simulink model "Trajectory"  (R2025a)
settings: Solver=VariableStepAuto  StartTime=0.0  StopTime=65  FixedStep=0.01  RelTol=1e-3
values from neighbouring files (symbols this model uses):
  L = 0.2    [untitled2.m]
  P = densifyPath(path, 0.05)    [untitled2.m]
  start = [1 1]    [untitled2.m]
undefined symbols (not defined in the file or in its folder): Actor, createShape
libraries: slpidlib x2, sim3dlib x2, robotalgslib x1
settings Model: Creator=mwali  LastModifiedBy=mwali

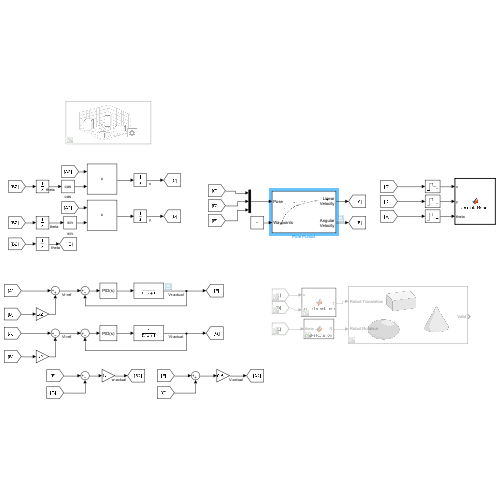
[thumbnail: Simulink's stored preview of the top-level diagram]
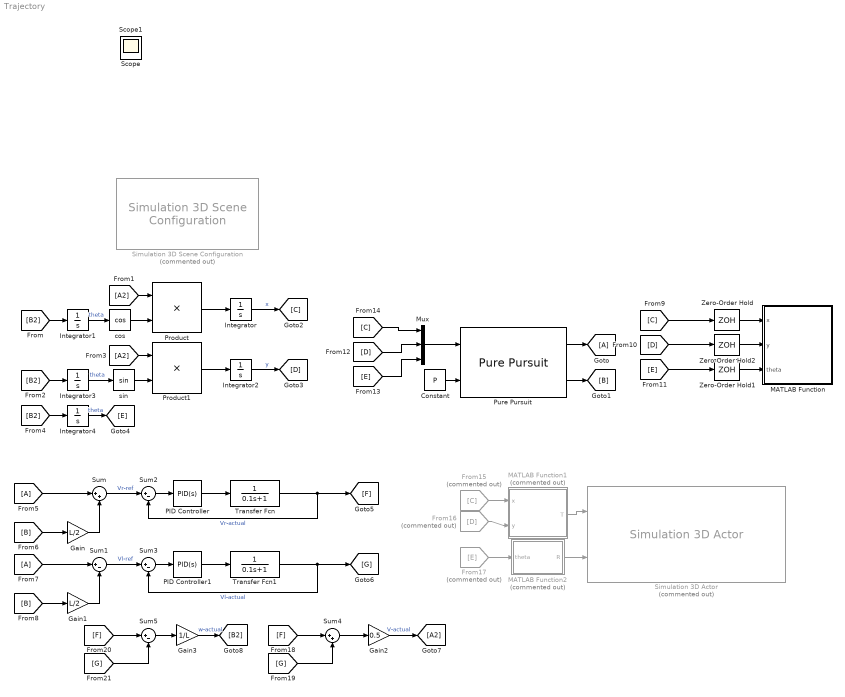
== system Trajectory ==
  Constant : Constant  Value=P
  From15 : From  Commented=on  GotoTag=C
  From16 : From  Commented=on  GotoTag=D
  From17 : From  Commented=on  GotoTag=E
  From5 : From
  From7 : From
  Gain : Gain  Gain=L/2
  Gain1 : Gain  Gain=L/2
  Gain2 : Gain  Gain=0.5
  Gain3 : Gain  Gain=1/L
  Goto : Goto
  Integrator : Integrator  InitialCondition=start(1)
  Integrator1 : Integrator
  Integrator2 : Integrator  InitialCondition=start(2)
  Integrator3 : Integrator
  Integrator4 : Integrator
  MATLAB Function : MATLAB Function  TreatAsAtomicUnit=on
  MATLAB Function1 : MATLAB Function  Commented=on  TreatAsAtomicUnit=on
  MATLAB Function2 : MATLAB Function  Commented=on  TreatAsAtomicUnit=on
  Mux : Mux  Inputs=3
  PID Controller : slpidlib/PID Controller  Controller=PID  Form=Parallel  TimeDomain=Continuous-time  UseExternalTs=off  SampleTime=-1  IntegratorMethod=Forward Euler  FilterMethod=Forward Euler  ControllerParametersSource=internal  P=1.08351767141455  I=20.5811272107881  UseKiTs=off  D=-0.0128072394159001  UseExternalDerivativeSource=off  N=84.6019689511989  UseFilter=on  TunerSelectOption=Transfer Function Based (PID Tuner App)  InitialConditionSource=internal  InitialConditionForIntegrator=0  InitialConditionForFilter=0  DifferentiatorICPrevScaledInput=0  ExternalReset=none  TrackingMode=off  Kt=1  LimitOutput=off  SatLimitsSource=internal  UpperSaturationLimit=inf  LowerSaturationLimit=-inf  LinearizeAsGain=on  AntiWindupMode=none  Kb=1  LimitIntegrator=off  UpperIntegratorSaturationLimit=inf  LowerIntegratorSaturationLimit=-inf  POutMin=[]  POutMax=[]  IOutMin=[]  IOutMax=[]  DOutMin=[]  DOutMax=[]  NOutMin=[]  NOutMax=[]  SumOutMin=[]  SumOutMax=[]  SaturationOutMin=[]  SaturationOutMax=[]  PParamMin=[]  PParamMax=[]  IParamMin=[]  IParamMax=[]  DParamMin=[]  DParamMax=[]  NParamMin=[]  NParamMax=[]  KbParamMin=[]  KbParamMax=[]  KtParamMin=[]  KtParamMax=[]  KbOutMin=[]  KbOutMax=[]  KtOutMin=[]  KtOutMax=[]  IntegratorOutMin=[]  IntegratorOutMax=[]  FilterOutMin=[]  FilterOutMax=[]  SumI1OutMin=[]  SumI1OutMax=[]  SumI2OutMin=[]  SumI2OutMax=[]  SumI3OutMin=[]  SumI3OutMax=[]  SumI4OutMin=[]  SumI4OutMax=[]  SumDOutMin=[]  SumDOutMax=[]  DifferentiatorOutMin=[]  DifferentiatorOutMax=[]  FilterDiffOutCoefMin=[]  FilterDiffOutCoefMax=[]  ReciprocalOutMin=[]  ReciprocalOutMax=[]  SumDenOutMin=[]  SumDenOutMax=[]  SumNumOutMin=[]  SumNumOutMax=[]  DivideOutMin=[]  DivideOutMax=[]  UdiffTsProdOutMin=[]  UdiffTsProdOutMax=[]  NTsProdOutMin=[]  NTsProdOutMax=[]  UintegralTsProdOutMin=[]  UintegralTsProdOutMax=[]  UngainTsProdOutMin=[]  UngainTsProdOutMax=[]  ClampingZeroOutDataTypeStr=Inherit: Inherit via back propagation  ClampingZeroOutMin=[]  ClampingZeroOutMax=[]  FilterDenConstantOutDataTypeStr=Inherit: Inherit via back propagation  FilterDenConstantOutMin=[]  FilterDenConstantOutMax=[]  PCopyOutDataTypeStr=Inherit: Inherit via back propagation  PCopyOutMin=[]  PCopyOutMax=[]  NCopyOutDataTypeStr=Inherit: Inherit via back propagation  NCopyOutMin=[]  NCopyOutMax=[]  IntegratorContinuousStateAttributes=''  IntegratorStateMustResolveToSignalObject=off  IntegratorRTWStateStorageClass=Auto  FilterContinuousStateAttributes=''  FilterStateMustResolveToSignalObject=off  FilterRTWStateStorageClass=Auto  ParallelPVariant=InternalParameters  IdealPVariant=Disabled  IVariant=InternalParameters  DVariant=InternalParameters  IntegratorVariant=Continuous  SatVariant=Disabled  AWVariant=Passthrough  PCopyVariant=Disabled  TRVariant=Disabled  FdbkBlocksVariant=Forward  IdealPFdbkVariant=Disabled  SatFdbkVariant=Disabled  DerivativeFilterVariant=ContFilter  NVariant=InternalParameters  NCopyVariant=Disabled  FilterICVariant=InternalICsFilter  IntegratorICVariant=InternalICs  ExternalResetVariant=Disabled  TRSumVariant=Passthrough  SumFdbkVariant=Disabled  SumVariant=Sum_PID  TsampFilterVariant=InternalTs  TsampNgainVariant=Passthrough  TsampIntegralVariant=Disabled_SignalSpec  ExternalSaturationOutDataTypeStr=Inherit: Same as second input  DerivativeSourceVariant=ErrorSignal  PreIntVariant=InternalPreInt
  PID Controller1 : slpidlib/PID Controller  Controller=PID  Form=Parallel  TimeDomain=Continuous-time  UseExternalTs=off  SampleTime=-1  IntegratorMethod=Forward Euler  FilterMethod=Forward Euler  ControllerParametersSource=internal  P=1.08351767141455  I=20.5811272107881  UseKiTs=off  D=-0.0128072394159001  UseExternalDerivativeSource=off  N=84.6019689511989  UseFilter=on  TunerSelectOption=Transfer Function Based (PID Tuner App)  InitialConditionSource=internal  InitialConditionForIntegrator=0  InitialConditionForFilter=0  DifferentiatorICPrevScaledInput=0  ExternalReset=none  TrackingMode=off  Kt=1  LimitOutput=off  SatLimitsSource=internal  UpperSaturationLimit=inf  LowerSaturationLimit=-inf  LinearizeAsGain=on  AntiWindupMode=none  Kb=1  LimitIntegrator=off  UpperIntegratorSaturationLimit=inf  LowerIntegratorSaturationLimit=-inf  POutMin=[]  POutMax=[]  IOutMin=[]  IOutMax=[]  DOutMin=[]  DOutMax=[]  NOutMin=[]  NOutMax=[]  SumOutMin=[]  SumOutMax=[]  SaturationOutMin=[]  SaturationOutMax=[]  PParamMin=[]  PParamMax=[]  IParamMin=[]  IParamMax=[]  DParamMin=[]  DParamMax=[]  NParamMin=[]  NParamMax=[]  KbParamMin=[]  KbParamMax=[]  KtParamMin=[]  KtParamMax=[]  KbOutMin=[]  KbOutMax=[]  KtOutMin=[]  KtOutMax=[]  IntegratorOutMin=[]  IntegratorOutMax=[]  FilterOutMin=[]  FilterOutMax=[]  SumI1OutMin=[]  SumI1OutMax=[]  SumI2OutMin=[]  SumI2OutMax=[]  SumI3OutMin=[]  SumI3OutMax=[]  SumI4OutMin=[]  SumI4OutMax=[]  SumDOutMin=[]  SumDOutMax=[]  DifferentiatorOutMin=[]  DifferentiatorOutMax=[]  FilterDiffOutCoefMin=[]  FilterDiffOutCoefMax=[]  ReciprocalOutMin=[]  ReciprocalOutMax=[]  SumDenOutMin=[]  SumDenOutMax=[]  SumNumOutMin=[]  SumNumOutMax=[]  DivideOutMin=[]  DivideOutMax=[]  UdiffTsProdOutMin=[]  UdiffTsProdOutMax=[]  NTsProdOutMin=[]  NTsProdOutMax=[]  UintegralTsProdOutMin=[]  UintegralTsProdOutMax=[]  UngainTsProdOutMin=[]  UngainTsProdOutMax=[]  ClampingZeroOutDataTypeStr=Inherit: Inherit via back propagation  ClampingZeroOutMin=[]  ClampingZeroOutMax=[]  FilterDenConstantOutDataTypeStr=Inherit: Inherit via back propagation  FilterDenConstantOutMin=[]  FilterDenConstantOutMax=[]  PCopyOutDataTypeStr=Inherit: Inherit via back propagation  PCopyOutMin=[]  PCopyOutMax=[]  NCopyOutDataTypeStr=Inherit: Inherit via back propagation  NCopyOutMin=[]  NCopyOutMax=[]  IntegratorContinuousStateAttributes=''  IntegratorStateMustResolveToSignalObject=off  IntegratorRTWStateStorageClass=Auto  FilterContinuousStateAttributes=''  FilterStateMustResolveToSignalObject=off  FilterRTWStateStorageClass=Auto  ParallelPVariant=InternalParameters  IdealPVariant=Disabled  IVariant=InternalParameters  DVariant=InternalParameters  IntegratorVariant=Continuous  SatVariant=Disabled  AWVariant=Passthrough  PCopyVariant=Disabled  TRVariant=Disabled  FdbkBlocksVariant=Forward  IdealPFdbkVariant=Disabled  SatFdbkVariant=Disabled  DerivativeFilterVariant=ContFilter  NVariant=InternalParameters  NCopyVariant=Disabled  FilterICVariant=InternalICsFilter  IntegratorICVariant=InternalICs  ExternalResetVariant=Disabled  TRSumVariant=Passthrough  SumFdbkVariant=Disabled  SumVariant=Sum_PID  TsampFilterVariant=InternalTs  TsampNgainVariant=Passthrough  TsampIntegralVariant=Disabled_SignalSpec  ExternalSaturationOutDataTypeStr=Inherit: Same as second input  DerivativeSourceVariant=ErrorSignal  PreIntVariant=InternalPreInt
  Product : Product
  Product1 : Product
  Pure Pursuit : robotalgslib/Pure Pursuit  DesiredLinearVelocityPort=off  DesiredLinearVelocity=0.2  MaxAngularVelocity=1.0  LookaheadDistancePort=off  LookaheadDistance=0.4  TargetDirPort=off  SimulateUsing=Code generation
      settings: LibrarySourceBlock=robotmobilelib/Pure Pursuit
  Simulation 3D Actor : sim3dlib/Simulation 3D Actor  Priority=1  Commented=on  ActorName=Robot  ParentName=Scene Origin  Operation=Create at setup  InitScriptText=createShape(Actor,'Box',[0.2 0.2 0.05]);  SampleTime=-1  Translation=[3 2.75 -0.025]  Rotation=[0 0 1.5708]  Scale=[1 1 1]  InputsText=Robot.Translation Robot.Rotation  aMode=5  ActorTag=Robot  ActorType=Sim3dActor  ID=1
  Simulation 3D Scene Configuration : sim3dlib/Simulation 3D Scene Configuration  Priority=0  Commented=on  ProjectFormat=Default Scenes  SceneDesc=Empty scene  ProjectName=C:\Program Files\MATLAB\R2025a\toolbox\shared\sim3d_projects\automotive_project_windows\UE\WindowsNoEditor\VehicleSimulation.exe  ScenePath=/Game/Maps/EmptyScene  EnableOpenDRIVE=off  vehTagList={'Custom';'Scene Origin';'Sim3dActor1'}  vehTag=Scene Origin  AttachedCameraRelativeTranslation=[0 0 0]  FreeCameraDefaultInitialTranslation=[-6, 0, 2]  AttachedCameraRelativeRotation=[0 0 0]  FreeCameraDefaultInitialRotation=[0, -15, 0]  ViewpointName=Custom  FreeCameraInitialTranslation=[0 0 0]  ViewpointTranslation=[0 0 0]  FreeCameraInitialRotation=[0 0 0]  ViewpointRotation=[0 0 0]  OpVisEn=off  Ts=0.02  EnableWindow=on  EnableRemoteAccess=off  EnableWeather=off  SunAzimuth=90  SunAltitude=40.0  EnableGeospatialSun=off  Latitude=0  Longitude=0  Date=2023-01-01  Time=10:30:00  GeoTimeZone=-5.0  SunDaylightSaving=off  wind=1  clouds=10  EnableVolumetricClouds=off  CloudCoverage=0  CloudAltitude=6  fog=0  rain=0  RaindropsEffect=off  SnowDensity=0  EnableGeospatial=off  TilesetSource=Earth terrain  UseTrueOrigin=off  OriginHeight=200  OriginLatitude=40.744652  OriginLongitude=-73.988864  MapStyle=Aerial  AdditionalAssetIDs=[]  UseAdvancedSunSky=off  SolarTime=11  TimeZone=-5  Day=21  Month=9  Year=2022  UseDaylightSavingTime=on  DSTStartDay=10  DSTStartMonth=3  DSTEndDay=3  DSTEndMonth=11  DSTSwitchHour=2  sensorTag=MainCamera1  sensorId=1  sensorName=MainCamera1  mountLoc=Origin  offsetFlag=off  tmountOffset=[0, 0, 0]  rmountOffset=[0, 0, 0]  HorizontalResolution=1280  VerticalResolution=720  HorizontalFOV=60  mountPoint=[0 0 0]  mountOrientation=[0 0 0]  aMode=6  ID=1  GeoTrigger=Inactive  ViewNameList={'Custom'}  ViewTranslationList={'[0 0 0]'}  ViewRotationList={'[0 0 0]'}
      settings: LibrarySourceBlock=robotsim3dlib/Simulation 3D Scene Configuration
  Sum : Sum  Inputs=|++
  Sum{1..3,5} (4 alike) : Sum  Inputs=|+-
  Sum4 : Sum  Inputs=|++
  Transfer Fcn : TransferFcn  Denominator=[0.1 1]
  Transfer Fcn1 : TransferFcn  Denominator=[0.1 1]
  Zero-Order Hold : ZeroOrderHold  SampleTime=0.01
  Zero-Order Hold1 : ZeroOrderHold  SampleTime=0.01
  Zero-Order Hold2 : ZeroOrderHold  SampleTime=0.01
  cos : Trigonometry  Operator=cos
  sin : Trigonometry
  Scope : Scope
      settings: ActiveDisplayYMinimum=-0.037808986482854419  ActiveDisplayYMaximum=0.34028087834568982
  Scope1 : Scope
      settings: ActiveDisplayYMinimum=-1  ActiveDisplayYMaximum=1
  wires:
  Product/1 -> Integrator/1
  cos/1 -> Product/2
  Integrator1/1 -> cos/1  "theta"
  [B2] -> Integrator1/1
  [A2] -> Product/1
  Pure Pursuit/1 -> Goto/1
  Pure Pursuit/2 -> [B]
  sin/1 -> Product1/2
  [B2] -> Integrator3/1
  Product1/1 -> Integrator2/1
  [A2] -> Product1/1
  Integrator3/1 -> sin/1  "theta"
  [B2] -> Integrator4/1
  Mux/1 -> Pure Pursuit/1
  Constant/1 -> Pure Pursuit/2
  Zero-Order Hold/1 -> MATLAB Function/1(x)
  Zero-Order Hold2/1 -> MATLAB Function/2(y)
  Zero-Order Hold1/1 -> MATLAB Function/3(theta)
  [B] -> Gain/1
  From5/1 -> Sum/1
  Gain/1 -> Sum/2
  From7/1 -> Sum1/1
  Gain1/1 -> Sum1/2
  [B] -> Gain1/1
  MATLAB Function1/1(T) -> Simulation 3D Actor/1
  Integrator/1 -> [C]  "x"
  Integrator2/1 -> [D]  "y"
  Integrator4/1 -> [E]  "theta"
  [C] -> Zero-Order Hold/1
  [D] -> Zero-Order Hold2/1
  [E] -> Zero-Order Hold1/1
  [C] -> Mux/1
  [D] -> Mux/2
  [E] -> Mux/3
  From15/1 -> MATLAB Function1/1(x)
  From16/1 -> MATLAB Function1/2(y)
  MATLAB Function2/1(R) -> Simulation 3D Actor/2
  From17/1 -> MATLAB Function2/1(theta)
  Sum/1 -> Sum2/1  "Vr-ref"
  Sum2/1 -> PID Controller/1
  PID Controller/1 -> Transfer Fcn/1
  Transfer Fcn/1 -> [F], Sum2/2  "Vr-actual"
  Transfer Fcn1/1 -> Sum3/2, [G]  "Vl-actual"
  PID Controller1/1 -> Transfer Fcn1/1
  Sum3/1 -> PID Controller1/1
  Sum1/1 -> Sum3/1  "Vl-ref"
  [F] -> Sum4/1
  [G] -> Sum4/2
  Sum4/1 -> Gain2/1
  Gain2/1 -> [A2]  "V-actual"
  [F] -> Sum5/1
  [G] -> Sum5/2
  Sum5/1 -> Gain3/1
  Gain3/1 -> [B2]  "w-actual"

== matlab function Trajectory/MATLAB Function ==
  data: x input; y input; theta input
function animateRobot(x,y,theta)

persistent hFig hRobot hTrail X Y

% Initialize persistent variables
if isempty(hFig)
    
    hFig = figure('Name','Robot Animation');
    axis equal
    grid on
    hold on
    xlabel('X')
    ylabel('Y')

    % create robot arrow
    hRobot = quiver(x,y,cos(theta),sin(theta),0.5,'LineWidth',2);

    % create trajectory line
    hTrail = plot(x,y,'b-');

    X = x;
    Y = y;

else
    
    % update trajectory
    X(end+1) = x;
    Y(end+1) = y;

    set(hTrail,'XData',X,'YData',Y)

    % update robot direction
    set(hRobot,'XData',x,'YData',y,'UData',cos(theta),'VData',sin(theta))

    drawnow limitrate

end

== matlab function Trajectory/MATLAB Function2 ==
  data: theta input; R output
function R = makeRotation(theta)
R = [0 0 theta];

== matlab function Trajectory/MATLAB Function1 ==
  data: x input; T output; y input
function T = makeTranslation(x,y)
T = [x y 0];
